simulink model "Traffic_lights_stateflow"  (R2018b)
settings: Solver=VariableStepAuto  StartTime=0.0  StopTime=10.0  RelTol=1e-3
settings Model: Creator=Conan  LastModifiedBy=Conan

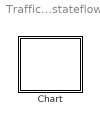
== system Traffic_lights_stateflow ==
  Chart : Stateflow chart  TreatAsAtomicUnit=on

== stateflow chart Traffic_lights_stateflow/Chart ==
  state State_of_Red
    en:
    Red_led = uint8(1);
    Yellow_led = uint8(0);
    Green_led = uint8(0);
    du:
    ex:
    Red_led = uint8(0);
    Yellow_led = uint8(0);
    Green_led = uint8(0);
  state State_of_yellow
    en:
    Red_led = uint8(0);
    Yellow_led = uint8(1);
    Green_led = uint8(0);
    du:
    ex:
    Red_led = uint8(0);
    Yellow_led = uint8(0);
    Green_led = uint8(0);
  state State_of_Green
    en:
    Red_led = uint8(0);
    Yellow_led =uint8(0);
    Green_led = uint8(1);
    du:
    ex:
    Red_led =  uint8(0);
    Yellow_led = uint8(0);
    Green_led = uint8(0);
  (default) -> State_of_Red
  State_of_Red -> State_of_yellow : [after(3,sec)]
  State_of_Green -> State_of_Red : [after(3,sec)]
  State_of_yellow -> State_of_Green : [after(3,sec)]
